simulink model "boiler_PSF_sim"  (R2020a)
settings: Solver=VariableStepAuto  StartTime=0.0  StopTime=tsim  MaxStep=0.001  RelTol=1e-3
values from neighbouring files (symbols this model uses):
  amppert = 0.2    [boiler_PSF.m]
  ampref = 1    [boiler_PSF.m]
  tpert = 40    [boiler_PSF.m]
  tref = 5    [boiler_PSF.m]
libraries: cstblocks x5
settings Model: Creator=treezao  LastModifiedBy=treezao

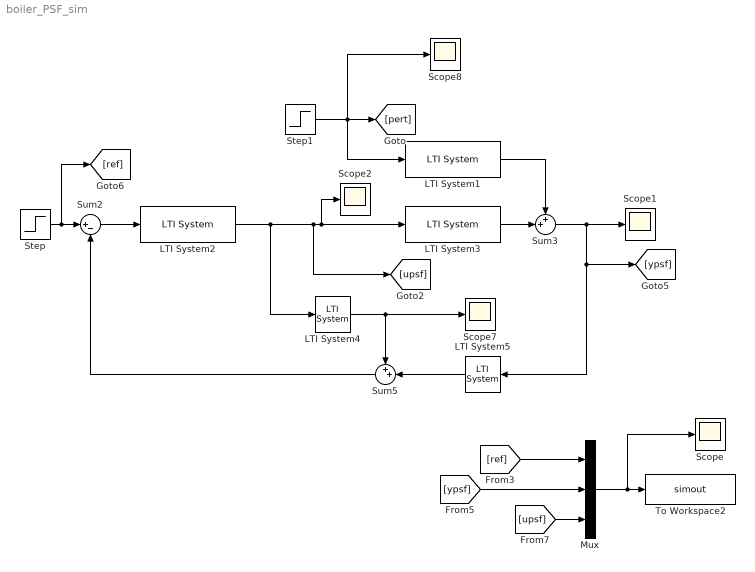
== system boiler_PSF_sim ==
  LTI System1 : cstblocks/LTI System  sys=Pq  IC=[]
  LTI System2 : cstblocks/LTI System  sys=Czps  IC=[]
  LTI System3 : cstblocks/LTI System  sys=P  IC=[]
  LTI System4 : cstblocks/LTI System  sys=Spsf  IC=[]
  LTI System5 : cstblocks/LTI System  sys=Fe  IC=[]
  Mux : Mux  Inputs=3
  Scope{,1..2,7..8} (5 alike) : Scope
  Step : Step  Time=tref  After=ampref  SampleTime=0
  Step1 : Step  Time=tpert  After=amppert  SampleTime=0
  Sum2 : Sum  Inputs=|+-
  Sum3 : Sum  Inputs=++|
  Sum5 : Sum  Inputs=++|
  To Workspace2 : ToWorkspace  VariableName=simout  SampleTime=-1
  wires:
  Sum2/1 -> LTI System2/1
  Step/1 -> [ref], Sum2/1
  LTI System2/1 -> Scope2/1, LTI System3/1, [upsf], LTI System4/1
  Step1/1 -> Scope8/1, LTI System1/1, [pert]
  Sum5/1 -> Sum2/2
  Mux/1 -> Scope/1, To Workspace2/1
  [ref] -> Mux/1
  [ypsf] -> Mux/2
  [upsf] -> Mux/3
  LTI System5/1 -> Sum5/2
  LTI System3/1 -> Sum3/2
  Sum3/1 -> [ypsf], LTI System5/1, Scope1/1
  LTI System1/1 -> Sum3/1
  LTI System4/1 -> Sum5/1, Scope7/1
